simulink library "navlib2"  (Simulink 3.00)
libraries: navlib2 x2
settings Model: LastModifiedBy=Dutchroll

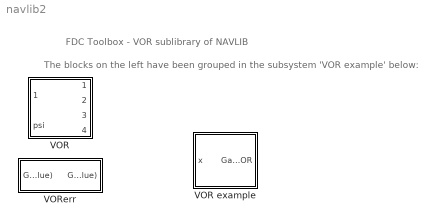
== system navlib2 ==
  note: FDC Toolbox - VOR sublibrary of NAVLIB
  note: The blocks on the left have been
      | grouped in the subsystem
      | 'VOR example' below:
  VOR : Subsystem  mask(VOR){xVOR=10000, yVOR=5000, HVOR=0, CD=0}
      mask prompts: xVOR "X-position of VOR station, relative to aircraft at t=0 sec. [m]:"; yVOR "Y-position of VOR station, relative to aircraft at t=0 sec. [m]:"; HVOR "Altitude of VOR station above sea level [m]:"; CD "Course Datum [deg]; 0 = north:"
      mask help: Calculation of nominal VOR signals
      mask init:
      | CD=CD*pi/180;
      mask Help: eval('fdchelp vor')
      mask Display: disp('Nominal\nVOR\nsignals')
  VOR example : Subsystem
      mask Display: plot(0,0,100,100,[86,85,90,86,80,85,0],[16,80,20,16,20,80,62],[22,18,25,28,22,19],[36,32,29,33,36,45],[17,15,12,18,16,19],[37,37,34,32,44,46],[22,31,47,52,19,15,28,22],[36,44,39,44,55,50,45,38],[31,28],[44,45],[20,18,17],[31,30,32],[36,35,36,37,36,35,35,35,33,31,25],[41,38,33,32,30,30,32,33,37,35,34],[85,42],[80,50],[86,87,87,86,84,83,84,85],[83,81,78,76,76,79,82,83])
  VORerr : Subsystem  mask(VOR error){@1=5}
      mask prompts: @1 "Overall VOR system error [%]:"
      mask help: Steady-state error VOR
      mask init:
      | KVORerr = 1 + (@1/100);
      mask Help: eval('browse vorerr')
      mask Display: disp('VOR Steady-\nstate error')

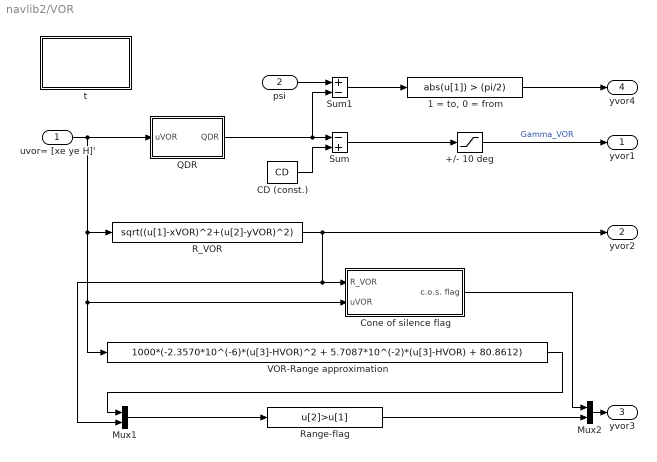
== system navlib2/VOR ==
  uvor= [xe ye H]' : Inport  Port=1  PortWidth=-1  SampleTime=-1  DataType=auto
      settings: SignalType=auto
  psi : Inport  Port=2  PortWidth=-1  SampleTime=-1  DataType=auto
      settings: SignalType=auto
  +/- 10 deg : Saturate  UpperLimit=10*pi/180  LowerLimit=-10*pi/180
  "1 = to, 0 = from" : Fcn  Expr=abs(u[1]) > (pi/2)
  CD (const.) : Constant  Value=CD
  Cone of silence flag : Subsystem
  Mux1 : Mux  Inputs=2
      settings: DisplayOption=none
  Mux2 : Mux  Inputs=2
      settings: DisplayOption=none
  QDR : Subsystem
  R_VOR : Fcn  Expr=sqrt((u[1]-xVOR)^2+(u[2]-yVOR)^2)
  Range-flag : Fcn  Expr=u[2]>u[1]
  Sum : Sum  Inputs=-+  SaturateOnIntegerOverflow=on
  Sum1 : Sum  Inputs=+-  SaturateOnIntegerOverflow=on
  VOR-Range approximation : Fcn  Expr=1000*(-2.3570*10^(-6)*(u[3]-HVOR)^2 + 5.7087*10^(-2)*(u[3]-HVOR) + 80.8612)
  t : Subsystem
      settings: OpenFcn=fdchelp vor
      mask Display: disp('VOR signals\nMarc Rauw\nJanuary 2005')
  yvor1 : Outport  Port=1
  yvor2 : Outport  Port=2
  yvor3 : Outport  Port=3
  yvor4 : Outport  Port=4
  wires:
  QDR/1(QDR) -> Sum1/2, Sum/1
  Cone of silence flag/1(c.o.s. flag) -> Mux2/1
  Mux2/1 -> yvor3/1
  VOR-Range approximation/1 -> Mux1/1
  Range-flag/1 -> Mux2/2
  Mux1/1 -> Range-flag/1
  R_VOR/1 -> Cone of silence flag/1(R_VOR), Mux1/2, yvor2/1
  Sum/1 -> +/- 10 deg/1
  +/- 10 deg/1 -> yvor1/1  "Gamma_VOR"
  Sum1/1 -> "1 = to, 0 = from"/1
  psi/1 -> Sum1/1
  CD (const.)/1 -> Sum/2
  "1 = to, 0 = from"/1 -> yvor4/1
  uvor= [xe ye H]'/1 -> QDR/1(uVOR), Cone of silence flag/2(uVOR), VOR-Range approximation/1, R_VOR/1

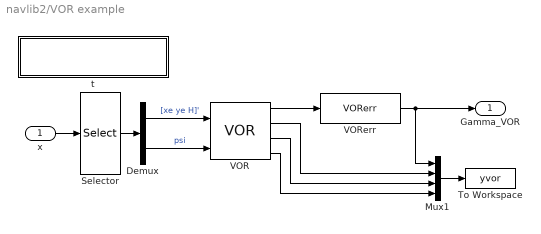
== system navlib2/VOR example ==
  x : Inport  Port=1  PortWidth=-1  SampleTime=-1  DataType=auto
      settings: SignalType=auto
  Demux : Demux  Outputs=[3 1]
  Mux1 : Mux  Inputs=[1 1 2 1]
      settings: DisplayOption=none
  Selector : Selector  Elements=[10 11 12 7]  InputPortWidth=12
  To Workspace : ToWorkspace  VariableName=yvor  SampleTime=0  SaveFormat=Matrix
      settings: Buffer=5000
  VOR : navlib2/VOR  xVOR=10000  yVOR=5000  HVOR=0  CD=0
  VORerr : navlib2/VORerr  MaskParam1=5
  t : Subsystem
      settings: OpenFcn=browse vorxmpl
      mask Display: disp('VOR example\nMarc Rauw, January 2005')
  Gamma_VOR : Outport  Port=1
  wires:
  VOR/1 -> VORerr/1
  Mux1/1 -> To Workspace/1
  VOR/2 -> Mux1/2
  VOR/3 -> Mux1/3
  VOR/4 -> Mux1/4
  VORerr/1 -> Gamma_VOR/1, Mux1/1
  x/1 -> Selector/1
  Selector/1 -> Demux/1
  Demux/1 -> VOR/1  "[xe ye H]'"
  Demux/2 -> VOR/2  "psi"

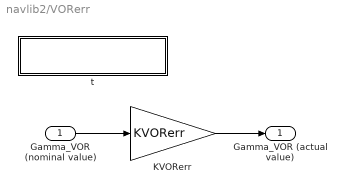
== system navlib2/VORerr ==
  Gamma_VOR (nominal value) : Inport  Port=1  PortWidth=-1  SampleTime=-1  DataType=auto
      settings: SignalType=auto
  KVORerr : Gain  Gain=KVORerr  SaturateOnIntegerOverflow=on
  t : Subsystem
      settings: OpenFcn=browse vorerr
      mask Display: disp('VOR steady-state error\nMarc Rauw, April 2003')
  Gamma_VOR (actual value) : Outport  Port=1
  wires:
  KVORerr/1 -> Gamma_VOR (actual value)/1
  Gamma_VOR (nominal value)/1 -> KVORerr/1

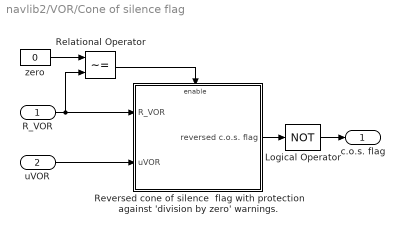
== system navlib2/VOR/Cone of silence flag ==
  R_VOR : Inport  Port=1  PortWidth=-1  SampleTime=-1  DataType=auto
      settings: SignalType=auto
  uVOR : Inport  Port=2  PortWidth=-1  SampleTime=-1  DataType=auto
      settings: SignalType=auto
  Logical Operator : Logic  Operator=NOT  Inputs=1
  Relational Operator : RelationalOperator  Operator=~=
  Reversed cone of silence  flag with protection against 'division by zero' warnings. : Subsystem
  zero : Constant  Value=0
  c.o.s. flag : Outport  Port=1
  wires:
  Reversed cone of silence  flag with protection against 'division by zero' warnings./1(reversed c.o.s. flag) -> Logical Operator/1
  uVOR/1 -> Reversed cone of silence  flag with protection against 'division by zero' warnings./2(uVOR)
  zero/1 -> Relational Operator/1
  R_VOR/1 -> Reversed cone of silence  flag with protection against 'division by zero' warnings./1(R_VOR), Relational Operator/2
  Relational Operator/1 -> Reversed cone of silence  flag with protection against 'division by zero' warnings./Enable
  Logical Operator/1 -> c.o.s. flag/1

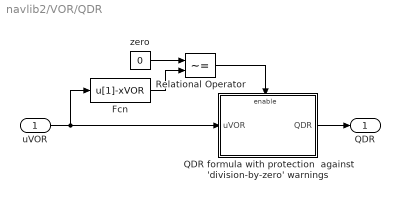
== system navlib2/VOR/QDR ==
  uVOR : Inport  Port=1  PortWidth=-1  SampleTime=-1  DataType=auto
      settings: SignalType=auto
  Fcn : Fcn  Expr=u[1]-xVOR
  QDR formula with protection  against 'division-by-zero' warnings : Subsystem
  Relational Operator : RelationalOperator  Operator=~=
  zero : Constant  Value=0
  QDR : Outport  Port=1
  wires:
  QDR formula with protection  against 'division-by-zero' warnings/1(QDR) -> QDR/1
  zero/1 -> Relational Operator/1
  Fcn/1 -> Relational Operator/2
  uVOR/1 -> QDR formula with protection  against 'division-by-zero' warnings/1(uVOR), Fcn/1
  Relational Operator/1 -> QDR formula with protection  against 'division-by-zero' warnings/Enable

== system navlib2/VOR/t ==

== system navlib2/VOR example/t ==

== system navlib2/VORerr/t ==

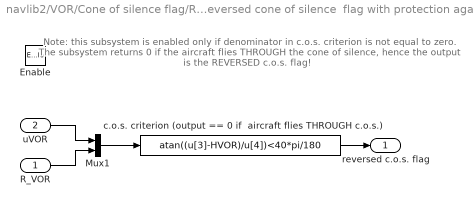
== system navlib2/VOR/Cone of silence flag/Reversed cone of silence  flag with protection against 'division by zero' warnings. ==
  note: Note: this subsystem is enabled only if denominator in c.o.s. criterion is
      | not equal to zero. The subsystem returns 0 if the aircraft flies THROUGH
      | the cone of silence, hence the output is the REVERSED c.o.s. flag!
  R_VOR : Inport  Port=1  PortWidth=-1  SampleTime=-1  DataType=auto
      settings: SignalType=auto
  uVOR : Inport  Port=2  PortWidth=-1  SampleTime=-1  DataType=auto
      settings: SignalType=auto
  Enable : EnablePort
  Mux1 : Mux  Inputs=[3 1]
      settings: DisplayOption=none
  c.o.s. criterion (output == 0 if  aircraft flies THROUGH c.o.s.) : Fcn  Expr=atan((u[3]-HVOR)/u[4])<40*pi/180
  reversed c.o.s. flag : Outport  Port=1  OutputWhenDisabled=reset  InitialOutput=0
  wires:
  uVOR/1 -> Mux1/1
  R_VOR/1 -> Mux1/2
  c.o.s. criterion (output == 0 if  aircraft flies THROUGH c.o.s.)/1 -> reversed c.o.s. flag/1
  Mux1/1 -> c.o.s. criterion (output == 0 if  aircraft flies THROUGH c.o.s.)/1

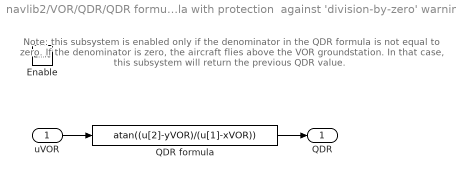
== system navlib2/VOR/QDR/QDR formula with protection  against 'division-by-zero' warnings ==
  note: Note: this subsystem is enabled only if the denominator in the
      | QDR formula is not equal to zero. If the denominator is zero,
      | the aircraft flies above the VOR groundstation. In that case,
      | this subsystem will return the previous QDR value.
  uVOR : Inport  Port=1  PortWidth=-1  SampleTime=-1  DataType=auto
      settings: SignalType=auto
  Enable : EnablePort
  QDR formula : Fcn  Expr=atan((u[2]-yVOR)/(u[1]-xVOR))
  QDR : Outport  Port=1  InitialOutput=0
  wires:
  uVOR/1 -> QDR formula/1
  QDR formula/1 -> QDR/1
